simulink library "Lib_LongPRACH"  (R2023b)
settings: Solver=VariableStepAuto  StartTime=0.0  StopTime=10.0  RelTol=1e-3
values from neighbouring files (symbols this model uses):
  prach = waveconfig.PRACH.Config    [hNRPRACHWaveformGenerator.m]
undefined symbols (not defined in the file or in its folder): AdvDSPBChannelOutDisplay, AdvDSPBDMemDisplay, AdvDSPBInDisplay, AdvDSPBOutDisplay, dpoly, dspba, dspba_ChannelInVis, dspba_ChannelOutVis, dspba_internal_get_channel_ports, evalAionMaskParam, latency, latencyCorrection, NTxAnts, primtype, UseDontCare, value
libraries: DSPBAPrim x553, DSPBABase x32, DSPBAFilters x24, DSPBAControl x18, DSPBAModelBus x8, DSPBAWaveformSynth x4, DspbAdvFftLibrary x2, DSPBAUtilities x2
(part 2 of 8)

== system Lib_LongPRACH/prach_wrap/MUX_ConfigId ==
  din0 : Inport
  vin0 : Inport  Port=2  OutDataTypeStr=boolean
  chin0 : Inport  Port=3  OutDataTypeStr=uint8
  SFN : Inport  Port=4
  HFN : Inport  Port=5
  prach_config_index : Inport  Port=6
  4G Config Index : Subsystem
  5G Config Index paired : Subsystem  Commented=on
  5G Config Index unpaired : Subsystem
  And : DSPBAPrim/And  primtype=and  nInputs=2  nOutputs=1  omode=Inherit via internal rule  otype=sfix(16)  scale=2^-15  rndmethod=Unbiased  factor=1  satmethod=Symmetric  shift_vec=[0 1 2 -1]  value=0  inPortNames=[' '; ' '; ' '; ' '; ' '; ' '; ' '; ' '; ' '; ' '; ' '; ' '; ' '; ' '; ' '; ' '; ]  outPortNames=[' ']  dspbaimage=dspba_prim.svg  text=fprintf('&');  style=Optimised  visibilities=8+2  version=20211007
  BitCombine : DSPBAPrim/BitCombine  primtype=bitcombine  nInputs=2  nOutputs=1  omode=Inherit via internal rule  otype=sfix(16)  scale=2^-15  rndmethod=Unbiased  factor=1  satmethod=Symmetric  shift_vec=[0 1 2 -1]  value=0  inPortNames=['l'; 'h';]  outPortNames=[' ']  dspbaimage=dspba_prim.svg  text=fprintf('[h,l]');  style=Optimised  visibilities=8+2  version=20211007
  ChannelIn : DSPBAPrim/ChannelIn  primtype=channelin  nInputs=dspba_internal_get_channel_ports(gcb)  nOutputs=dspba_internal_get_channel_ports(gcb)  omode=Inherit via internal rule  otype=sfix(16)  scale=2^-15  rndmethod=Unbiased  factor=1  satmethod=Symmetric  shift_vec=[0 1 2 -1]  value=1  inPortNames=['v'; 'c'; '0'; '1'; '2'; '3'; '4'; '5'; '6'; '7'; '8'; '9'; 'A'; 'B'; 'D'; 'E'; 'F'; 'G'; 'H'; 'I'; 'J'; 'K'; 'L'; 'M'; 'N'; 'O'; 'P'; 'Q'; 'R'; 'S'; 'T'; 'U'; 'W'; 'X'; 'Y'; 'Z']  outPortNames=['v'; 'c'; '0'; '1'; '2'; '3'; '4'; '5'; '6'; '7'; '8'; '9'; 'A'; 'B'; 'D'; 'E'; 'F'; 'G'; 'H'; 'I'; 'J'; 'K'; 'L'; 'M'; 'N'; 'O'; 'P'; 'Q'; 'R'; 'S'; 'T'; 'U'; 'W'; 'X'; 'Y'; 'Z']  dspbaimage=dspba_prim_channel_tall.svg  text=fprintf('In');  style=Optimised  dataSignals=1  foldingEnabled=off  channels=1  sampleRate=200  packetBeginPresent=off  packetBeginEnabled=off  visibilities=dspba_ChannelInVis(gcb)  latencyCorrection=0  scheduleOrigin=on  version=20211214
  ChannelOut : DSPBAPrim/ChannelOut  primtype=channelout  nInputs=dspba_internal_get_channel_ports(gcb)  nOutputs=dspba_internal_get_channel_ports(gcb)  omode=Inherit via internal rule  otype=sfix(16)  scale=2^-15  rndmethod=Unbiased  factor=1  satmethod=Symmetric  shift_vec=[0 1 2 -1]  value=2  inPortNames=['v'; 'c'; '0'; '1'; '2'; '3'; '4'; '5'; '6'; '7'; '8'; '9'; 'A'; 'B'; 'D'; 'E'; 'F'; 'G'; 'H'; 'I'; 'J'; 'K'; 'L'; 'M'; 'N'; 'O'; 'P'; 'Q'; 'R'; 'S'; 'T'; 'U'; 'W'; 'X'; 'Y'; 'Z']  outPortNames=['v'; 'c'; '0'; '1'; '2'; '3'; '4'; '5'; '6'; '7'; '8'; '9'; 'A'; 'B'; 'D'; 'E'; 'F'; 'G'; 'H'; 'I'; 'J'; 'K'; 'L'; 'M'; 'N'; 'O'; 'P'; 'Q'; 'R'; 'S'; 'T'; 'U'; 'W'; 'X'; 'Y'; 'Z']  dspbaimage=dspba_prim_channel_tall.svg  text=fprintf('Out%s', AdvDSPBChannelOutDisplay(latency));  style=Optimised  dataSignals=2  foldingEnabled=off  channels=1  sampleRate=200  packetBeginPresent=off  packetBeginEnabled=off  visibilities=dspba_ChannelOutVis(gcb)  latency=1  latencyCorrection=0  version=20211214
  Convert2 : DSPBAPrim/Convert  primtype=convert  nInputs=1  nOutputs=1  omode=Specify via dialog  otype=uint(4)  scale=2^0  rndmethod=Truncate  factor=1  satmethod=None  shift_vec=[0 1 2 -1]  value=round([0:255]/17)  inPortNames=[' '; ' ';]  outPortNames=[' '; 'c']  dspbaimage=dspba_prim_wide.svg  text=fprintf('convert');  style=Optimised  visibilities=8+64+256+2^17  clipdetect=off  floatPrecision=float32_m23  advOptions=[]  version=20211007
  GPIn : DSPBAPrim/GPIn  primtype=gpin  nInputs=evalAionMaskParam(gcb,'value',1)  nOutputs=evalAionMaskParam(gcb,'value',1)  omode=Inherit via internal rule  otype=sfix(16)  scale=2^-15  rndmethod=Unbiased  factor=1  satmethod=Symmetric  shift_vec=[0 1 2 -1]  value=1  inPortNames=[' ' ' ' ' ' ' ' ' ' ' ' ' ' ' ' ' ' ' ' ' ' ' ' ' ' ' ' ' ' ' ' ' ' ' ' ' ' ' ' ' ' ' ' ' ' ' ' ' ' ' ' ' ' ' ' ' ' ' ' ' ' ' ' ' ' ' ' ' ']'  outPortNames=[' ' ' ' ' ' ' ' ' ' ' ' ' ' ' ' ' ' ' ' ' ' ' ' ' ' ' ' ' ' ' ' ' ' ' ' ' ' ' ' ' ' ' ' ' ' ' ' ' ' ' ' ' ' ' ' ' ' ' ' ' ' ' ' ' ' ' ' ' ']'  dspbaimage=dspba_prim_channel_tall.svg  text=fprintf('GPIn');  style=Optimised  visibilities=1024  latencyCorrection=0  scheduleOrigin=on  version=20211214
  GPIn1 : DSPBAPrim/GPIn  primtype=gpin  nInputs=evalAionMaskParam(gcb,'value',1)  nOutputs=evalAionMaskParam(gcb,'value',1)  omode=Inherit via internal rule  otype=sfix(16)  scale=2^-15  rndmethod=Unbiased  factor=1  satmethod=Symmetric  shift_vec=[0 1 2 -1]  value=1  inPortNames=[' ' ' ' ' ' ' ' ' ' ' ' ' ' ' ' ' ' ' ' ' ' ' ' ' ' ' ' ' ' ' ' ' ' ' ' ' ' ' ' ' ' ' ' ' ' ' ' ' ' ' ' ' ' ' ' ' ' ' ' ' ' ' ' ' ' ' ' ' ']'  outPortNames=[' ' ' ' ' ' ' ' ' ' ' ' ' ' ' ' ' ' ' ' ' ' ' ' ' ' ' ' ' ' ' ' ' ' ' ' ' ' ' ' ' ' ' ' ' ' ' ' ' ' ' ' ' ' ' ' ' ' ' ' ' ' ' ' ' ' ' ' ' ']'  dspbaimage=dspba_prim_channel_tall.svg  text=fprintf('GPIn');  style=Optimised  visibilities=1024  latencyCorrection=0  scheduleOrigin=on  version=20211214
  GPIn2 : DSPBAPrim/GPIn  primtype=gpin  nInputs=evalAionMaskParam(gcb,'value',1)  nOutputs=evalAionMaskParam(gcb,'value',1)  omode=Inherit via internal rule  otype=sfix(16)  scale=2^-15  rndmethod=Unbiased  factor=1  satmethod=Symmetric  shift_vec=[0 1 2 -1]  value=1  inPortNames=[' ' ' ' ' ' ' ' ' ' ' ' ' ' ' ' ' ' ' ' ' ' ' ' ' ' ' ' ' ' ' ' ' ' ' ' ' ' ' ' ' ' ' ' ' ' ' ' ' ' ' ' ' ' ' ' ' ' ' ' ' ' ' ' ' ' ' ' ' ']'  outPortNames=[' ' ' ' ' ' ' ' ' ' ' ' ' ' ' ' ' ' ' ' ' ' ' ' ' ' ' ' ' ' ' ' ' ' ' ' ' ' ' ' ' ' ' ' ' ' ' ' ' ' ' ' ' ' ' ' ' ' ' ' ' ' ' ' ' ' ' ' ' ']'  dspbaimage=dspba_prim_channel_tall.svg  text=fprintf('GPIn');  style=Optimised  visibilities=1024  latencyCorrection=0  scheduleOrigin=on  version=20211214
  Mux1 : DSPBAPrim/Mux  primtype=mux  nInputs=evalAionMaskParam(gcb,'value',1)+1  nOutputs=1  omode=Inherit via internal rule  otype=sfix(16)  scale=2^-15  rndmethod=Unbiased  factor=1  satmethod=Symmetric  shift_vec=[0 1 2 -1]  value=2  inPortNames=['s '; 'd0'; 'd1'; 'd2'; 'd3'; 'd4'; 'd5'; 'd6'; 'd7'; 'd8'; 'd9';]  outPortNames=[' ']  dspbaimage=dspba_prim_tall.svg  text=fprintf('%s', primtype);  style=Optimised  visibilities=1032  version=20211007
  RegField2 : DSPBAModelBus/RegField  reg_name=MMoffset.prach_technology  reg_rwmode=Read/Write  reg_msb=0  reg_lsb=0  reg_mode=Specify via dialog  reg_type=ufix(1)  reg_scale=2^0  reg_init=prach_technology  reg_desc=4G = 0, 5G = 1 Technology  reg_modal=off  reg_desc0=0  reg_desc1=0  reg_desc2=0  reg_desc3=0  reg_desc4=0  reg_desc5=0  reg_desc6=0  reg_desc7=0  SampleTime=-1  version=20090407
  SynthesisInfo : DSPBAPrim/SynthesisInfo  primtype=synthinfo  nInputs=0  nOutputs=0  omode=Inherit via internal rule  otype=sfix(16)  scale=2^-15  rndmethod=Truncate  factor=1  satmethod=Symmetric  shift_vec=[0 1 2 -1]  value=99  inPortNames=[' '; ' ';]  outPortNames=[' ']  dspbaimage=dspba_prim_ctrl.jpg  text=fprintf('Style=%s', style);  style=Scheduled  visibilities=2^17+2^18+2^19+2^20+2^21+2^22+2^23+2^24  constraintPair=None  constraintRelation=>  constraintLimit=2  modelRefSign=+  modelRef=''  showSchedule=off  simulationMode=Use Global Value  resetMinimization=Conditional - On for ChannelIn/Out only  version=20220106
  dout : Outport  VectorParamsAs1DForOutWhenUnconnected=off
  vout : Outport  Port=2  VectorParamsAs1DForOutWhenUnconnected=off
  cout : Outport  Port=3  VectorParamsAs1DForOutWhenUnconnected=off
  TimeReference : Outport  Port=4  VectorParamsAs1DForOutWhenUnconnected=off
  wires:
  ChannelIn/1 -> And/2
  ChannelOut/1 -> vout/1
  ChannelOut/2 -> cout/1
  ChannelOut/3 -> dout/1
  ChannelIn/2 -> ChannelOut/2
  And/1 -> ChannelOut/1
  SFN/1 -> GPIn1/1
  HFN/1 -> GPIn/1
  prach_config_index/1 -> GPIn2/1
  vin0/1 -> ChannelIn/1
  chin0/1 -> ChannelIn/2
  din0/1 -> ChannelIn/3
  ChannelIn/3 -> ChannelOut/3
  GPIn/1 -> Convert2/1
  Convert2/1 -> BitCombine/1, 5G Config Index unpaired/1(SubFrame), 4G Config Index/3(SubFrame)
  GPIn2/1 -> 4G Config Index/1(ConfigIdx), 5G Config Index unpaired/2(ConfigIdx)
  GPIn1/1 -> BitCombine/2, 5G Config Index unpaired/3(SFN), 4G Config Index/2(SFN)
  5G Config Index unpaired/1(Out2) -> Mux1/3
  Mux1/1 -> And/1
  4G Config Index/1(Out2) -> Mux1/2
  RegField2/1 -> Mux1/1
  BitCombine/1 -> ChannelOut/4
  ChannelOut/4 -> TimeReference/1

== system Lib_LongPRACH/prach_wrap/S2B_FFT ==
  note: FFT
  note: scaling
  din : Inport
  vin : Inport  Port=2
  cin : Inport  Port=3
  Complex to Real-Imag : ComplexToRealImag
  Const6 : DSPBAPrim/Const  primtype=const  nInputs=0  nOutputs=1  omode=Inherit via back propagation  otype=ufix(8)  scale=2^0  rndmethod=Unbiased  factor=1  satmethod=Symmetric  shift_vec=[0 1 2 -1]  value=1  inPortNames=['+'; '+';]  outPortNames=[' ']  dspbaimage=dspba_prim.svg  text=fprintf('%s', num2str(value));  style=Optimised  visibilities=8 + 1024  floatPrecision=float32_m23  warnSaturation=on  version=20211007  SampleTime=inf
  FFT1 : DspbAdvFftLibrary/Common/FFT  IFFT=false  subchannels=1  br_in=true  N=nextpow2(prach.Nfft)  in_type=fixdt(1,16,15)  type_strings=dspba.fft.full_wordgrowth(true, false, nextpow2(prach.Nfft), fixdt(1,16,15), fixdt(1,16,15))  faithful=false
      link override ChannelOut1: nInputs=dspba_internal_get_channel_ports(gcb, 'inputs')  nOutputs=dspba_internal_get_channel_ports(gcb, 'outputs')  value=1  packetBeginEnabled=off  latency=57  version=20140818
  Real-Imag to Complex : RealImagToComplex
  RegField1 : DSPBAModelBus/RegField  Commented=on  reg_name=MMoffset.prach_fft_scale  reg_rwmode=Read/Write  reg_msb=5  reg_lsb=0  reg_mode=Specify via dialog  reg_type=ufix(6)  reg_scale=2^0  reg_init=18  reg_desc=PRACH Sym Extraction Registers  reg_modal=off  reg_desc0=0  reg_desc1=0  reg_desc2=0  reg_desc3=0  reg_desc4=0  reg_desc5=0  reg_desc6=0  reg_desc7=0  SampleTime=-1  version=20090407
  S2B : Subsystem
  Scale : DSPBABase/Scale  otype=sfix(16)  scale=2^-FFT_frac_scaling  rndmethod=Biased  factor=1  satmethod=Symmetric  shift_vec=0  latency=3  simulationMode=Use Global Value  version=20130807
  Scale1 : DSPBABase/Scale  otype=sfix(16)  scale=2^-FFT_frac_scaling  rndmethod=Biased  factor=1  satmethod=Symmetric  shift_vec=0  latency=3  simulationMode=Use Global Value  version=20130807
  Terminator{,1..3} (4 alike) : Terminator
  To Workspace1 : ToWorkspace  VariableName=S2B_dout  SampleTime=-1
  To Workspace2 : ToWorkspace  VariableName=S2B_valid  SampleTime=-1
  To Workspace3 : ToWorkspace  VariableName=S2B_chout  SampleTime=-1
  To Workspace4 : ToWorkspace  VariableName=fftcore_vout  SampleTime=-1
  To Workspace5 : ToWorkspace  VariableName=fftcore_chout  SampleTime=-1
  To Workspace6 : ToWorkspace  VariableName=fftcore_dout  SampleTime=-1
  dout : Outport  VectorParamsAs1DForOutWhenUnconnected=off
  vout : Outport  Port=2  VectorParamsAs1DForOutWhenUnconnected=off
  cout : Outport  Port=3  VectorParamsAs1DForOutWhenUnconnected=off
  wires:
  Real-Imag to Complex/1 -> dout/1
  Scale/2 -> vout/1
  Scale/3 -> cout/1
  din/1 -> S2B/1(data_in)
  vin/1 -> S2B/2(data_valid)
  Scale/4 -> Terminator3/1
  Const6/1 -> Scale/4, Scale1/4
  Scale1/4 -> Terminator2/1
  Scale1/3 -> Terminator1/1
  Scale1/2 -> Terminator/1
  Scale1/1 -> Real-Imag to Complex/2
  FFT1/2 -> To Workspace5/1, Scale/3, Scale1/3
  FFT1/3 -> To Workspace6/1, Complex to Real-Imag/1
  Complex to Real-Imag/2 -> Scale1/1
  Scale/1 -> Real-Imag to Complex/1
  Complex to Real-Imag/1 -> Scale/1
  FFT1/1 -> To Workspace4/1, Scale1/2, Scale/2
  S2B/3(ch_no) -> FFT1/2, To Workspace3/1
  S2B/2(valid_out) -> To Workspace2/1, FFT1/1
  S2B/1(data_out) -> To Workspace1/1, FFT1/3
  cin/1 -> S2B/3(chin)

== system Lib_LongPRACH/prach_wrap/SYM_SELECT ==
  note: rising edge dv required TBD??
  note: prach start point tbd
  din : Inport
  vin : Inport  Port=2
  chin : Inport  Port=3
  TimeRef : Inport  Port=4
  And : DSPBAPrim/And  primtype=and  nInputs=2  nOutputs=1  omode=Inherit via internal rule  otype=sfix(16)  scale=2^-15  rndmethod=Unbiased  factor=1  satmethod=Symmetric  shift_vec=[0 1 2 -1]  value=0  inPortNames=[' '; ' '; ' '; ' '; ' '; ' '; ' '; ' '; ' '; ' '; ' '; ' '; ' '; ' '; ' '; ' '; ]  outPortNames=[' ']  dspbaimage=dspba_prim.svg  text=fprintf('&');  style=Optimised  visibilities=8+2  version=20211007
  And1 : DSPBAPrim/And  primtype=and  nInputs=2  nOutputs=1  omode=Inherit via internal rule  otype=sfix(16)  scale=2^-15  rndmethod=Unbiased  factor=1  satmethod=Symmetric  shift_vec=[0 1 2 -1]  value=0  inPortNames=[' '; ' '; ' '; ' '; ' '; ' '; ' '; ' '; ' '; ' '; ' '; ' '; ' '; ' '; ' '; ' '; ]  outPortNames=[' ']  dspbaimage=dspba_prim.svg  text=fprintf('&');  style=Optimised  visibilities=8+2  version=20211007
  And2 : DSPBAPrim/And  primtype=and  nInputs=2  nOutputs=1  omode=Inherit via internal rule  otype=sfix(16)  scale=2^-15  rndmethod=Unbiased  factor=1  satmethod=Symmetric  shift_vec=[0 1 2 -1]  value=0  inPortNames=[' '; ' '; ' '; ' '; ' '; ' '; ' '; ' '; ' '; ' '; ' '; ' '; ' '; ' '; ' '; ' '; ]  outPortNames=[' ']  dspbaimage=dspba_prim.svg  text=fprintf('&');  style=Optimised  visibilities=8+2  version=20211007
  ChannelIn : DSPBAPrim/ChannelIn  primtype=channelin  nInputs=dspba_internal_get_channel_ports(gcb)  nOutputs=dspba_internal_get_channel_ports(gcb)  omode=Inherit via internal rule  otype=sfix(16)  scale=2^-15  rndmethod=Unbiased  factor=1  satmethod=Symmetric  shift_vec=[0 1 2 -1]  value=2  inPortNames=['v'; 'c'; '0'; '1'; '2'; '3'; '4'; '5'; '6'; '7'; '8'; '9'; 'A'; 'B'; 'D'; 'E'; 'F'; 'G'; 'H'; 'I'; 'J'; 'K'; 'L'; 'M'; 'N'; 'O'; 'P'; 'Q'; 'R'; 'S'; 'T'; 'U'; 'W'; 'X'; 'Y'; 'Z']  outPortNames=['v'; 'c'; '0'; '1'; '2'; '3'; '4'; '5'; '6'; '7'; '8'; '9'; 'A'; 'B'; 'D'; 'E'; 'F'; 'G'; 'H'; 'I'; 'J'; 'K'; 'L'; 'M'; 'N'; 'O'; 'P'; 'Q'; 'R'; 'S'; 'T'; 'U'; 'W'; 'X'; 'Y'; 'Z']  dspbaimage=dspba_prim_channel_tall.svg  text=fprintf('In');  style=Optimised  dataSignals=2  foldingEnabled=off  channels=1  sampleRate=200  packetBeginPresent=off  packetBeginEnabled=off  visibilities=dspba_ChannelInVis(gcb)  latencyCorrection=0  scheduleOrigin=on  version=20211214
  ChannelOut : DSPBAPrim/ChannelOut  primtype=channelout  nInputs=dspba_internal_get_channel_ports(gcb)  nOutputs=dspba_internal_get_channel_ports(gcb)  omode=Inherit via internal rule  otype=sfix(16)  scale=2^-15  rndmethod=Unbiased  factor=1  satmethod=Symmetric  shift_vec=[0 1 2 -1]  value=2  inPortNames=['v'; 'c'; '0'; '1'; '2'; '3'; '4'; '5'; '6'; '7'; '8'; '9'; 'A'; 'B'; 'D'; 'E'; 'F'; 'G'; 'H'; 'I'; 'J'; 'K'; 'L'; 'M'; 'N'; 'O'; 'P'; 'Q'; 'R'; 'S'; 'T'; 'U'; 'W'; 'X'; 'Y'; 'Z']  outPortNames=['v'; 'c'; '0'; '1'; '2'; '3'; '4'; '5'; '6'; '7'; '8'; '9'; 'A'; 'B'; 'D'; 'E'; 'F'; 'G'; 'H'; 'I'; 'J'; 'K'; 'L'; 'M'; 'N'; 'O'; 'P'; 'Q'; 'R'; 'S'; 'T'; 'U'; 'W'; 'X'; 'Y'; 'Z']  dspbaimage=dspba_prim_channel_tall.svg  text=fprintf('Out%s', AdvDSPBChannelOutDisplay(latency));  style=Optimised  dataSignals=2  foldingEnabled=off  channels=1  sampleRate=200  packetBeginPresent=off  packetBeginEnabled=off  visibilities=dspba_ChannelOutVis(gcb)  latency=3  latencyCorrection=0  version=20211214
  CmpEQ : DSPBAPrim/CmpEQ  primtype=cmpeq  nInputs=2  nOutputs=1  omode=boolean  otype=sfix(16)  scale=2^-15  rndmethod=Unbiased  factor=1  satmethod=Symmetric  shift_vec=[0 1 2 -1]  value=0  inPortNames=[' '; ' ';]  outPortNames=[' ']  dspbaimage=dspba_prim.svg  text=fprintf('==');  style=Optimised  visibilities=0  advOptions=[]  version=20211007
  CmpGE : DSPBAPrim/CmpGE  primtype=cmpgte  nInputs=2  nOutputs=1  omode=boolean  otype=sfix(16)  scale=2^-15  rndmethod=Unbiased  factor=1  satmethod=Symmetric  shift_vec=[0 1 2 -1]  value=0  inPortNames=['a'; 'b';]  outPortNames=[' ']  dspbaimage=dspba_prim.svg  text=fprintf('a>=b');  style=Optimised  visibilities=0  advOptions=[]  version=20211007
  CmpLT : DSPBAPrim/CmpLT  primtype=cmplt  nInputs=2  nOutputs=1  omode=boolean  otype=sfix(16)  scale=2^-15  rndmethod=Unbiased  factor=1  satmethod=Symmetric  shift_vec=[0 1 2 -1]  value=0  inPortNames=['a'; 'b';]  outPortNames=[' ']  dspbaimage=dspba_prim.svg  text=fprintf('a<b');  style=Optimised  visibilities=0  advOptions=[]  version=20211007
  Const2 : DSPBAPrim/Const  primtype=const  nInputs=0  nOutputs=1  omode=Specify via dialog  otype=ufix(1)  scale=2^-0  rndmethod=Unbiased  factor=1  satmethod=Symmetric  shift_vec=[0 1 2 -1]  value=0  inPortNames=['+'; '+';]  outPortNames=[' ']  dspbaimage=dspba_prim.svg  text=fprintf('%s', num2str(value));  style=Optimised  visibilities=8 + 1024  floatPrecision=float32_m23  warnSaturation=on  version=20211007  SampleTime=inf
  Counter : DSPBAPrim/Counter  primtype=counter  nInputs=1  nOutputs=1  omode=Inherit via internal rule  otype=ufix(16)  scale=2^-0  rndmethod=Unbiased  factor=1  satmethod=Symmetric  shift_vec=[0 1 2 -1]  value=[prach.Nfft-1 prach.Nfft 1]  inPortNames=[' '; ' ';]  outPortNames=[' ']  dspbaimage=dspba_prim.svg  text=fprintf('counter\n[%d %d %d]', value(1), value(2), value(3));  style=Optimised  visibilities=8 + 1024  version=20211007
  RegField1 : DSPBAModelBus/RegField  reg_name=MMoffset.prach_out_start  reg_rwmode=Read/Write  reg_msb=15  reg_lsb=0  reg_mode=Specify via dialog  reg_type=ufix(16)  reg_scale=2^0  reg_init=prach.SCstart-1  reg_desc=PRACH Sym Extraction Registers  reg_modal=off  reg_desc0=0  reg_desc1=0  reg_desc2=0  reg_desc3=0  reg_desc4=0  reg_desc5=0  reg_desc6=0  reg_desc7=0  SampleTime=-1  version=20090407
  RegField2 : DSPBAModelBus/RegField  reg_name=MMoffset.prach_out_end  reg_rwmode=Read/Write  reg_msb=15  reg_lsb=0  reg_mode=Specify via dialog  reg_type=ufix(16)  reg_scale=2^0  reg_init=prach.SCend  reg_desc=PRACH Sym Extraction Registers  reg_modal=off  reg_desc0=0  reg_desc1=0  reg_desc2=0  reg_desc3=0  reg_desc4=0  reg_desc5=0  reg_desc6=0  reg_desc7=0  SampleTime=-1  version=20090407
  SynthesisInfo : DSPBAPrim/SynthesisInfo  primtype=synthinfo  nInputs=0  nOutputs=0  omode=Inherit via internal rule  otype=sfix(16)  scale=2^-15  rndmethod=Truncate  factor=1  satmethod=Symmetric  shift_vec=[0 1 2 -1]  value=99  inPortNames=[' '; ' ';]  outPortNames=[' ']  dspbaimage=dspba_prim_ctrl.jpg  text=fprintf('Style=%s', style);  style=Scheduled  visibilities=2^17+2^18+2^19+2^20+2^21+2^22+2^23+2^24  constraintPair=None  constraintRelation=>  constraintLimit=2  modelRefSign=+  modelRef=''  showSchedule=off  simulationMode=Use Global Value  resetMinimization=Conditional - On for ChannelIn/Out only  version=20220106
  To Workspace12 : ToWorkspace  VariableName=prach_cout  SampleTime=-1
  To Workspace7 : ToWorkspace  VariableName=prach_vout  SampleTime=-1
  To Workspace8 : ToWorkspace  VariableName=prach_dout  SampleTime=-1
  Zero_insertion : Subsystem
  latch_0L : DSPBAControl/latch_0L
  dout : Outport  VectorParamsAs1DForOutWhenUnconnected=off
  vout : Outport  Port=2  VectorParamsAs1DForOutWhenUnconnected=off
  cout : Outport  Port=3  VectorParamsAs1DForOutWhenUnconnected=off
  TimeReference : Outport  Port=4  VectorParamsAs1DForOutWhenUnconnected=off
  wires:
  RegField2/1 -> CmpLT/2
  RegField1/1 -> CmpGE/2
  Counter/1 -> CmpLT/1, CmpGE/1
  ChannelIn/1 -> And/1, Counter/1
  ChannelOut/1 -> To Workspace7/1, vout/1
  ChannelOut/2 -> To Workspace12/1, cout/1
  ChannelOut/3 -> dout/1, To Workspace8/1
  din/1 -> ChannelIn/3
  chin/1 -> ChannelIn/2
  vin/1 -> ChannelIn/1
  CmpGE/1 -> And2/1
  CmpLT/1 -> And2/2
  And2/1 -> And/2
  And/1 -> Zero_insertion/1(valid_in), And1/1
  TimeRef/1 -> ChannelIn/4
  ChannelOut/4 -> TimeReference/1
  ChannelIn/4 -> latch_0L/2
  ChannelIn/2 -> Zero_insertion/2(chin), CmpEQ/1
  Const2/1 -> CmpEQ/2
  CmpEQ/1 -> And1/2
  And1/1 -> latch_0L/1
  latch_0L/1 -> ChannelOut/4
  Zero_insertion/3(dataout) -> ChannelOut/3
  Zero_insertion/1(valid_out) -> ChannelOut/1
  Zero_insertion/2("chout ") -> ChannelOut/2
  ChannelIn/3 -> Zero_insertion/3(datain)

== system Lib_LongPRACH/Longprach_C_M_plane/LongPRACH_core/CP_REMOVAL ==
  din : Inport
  vin : Inport  Port=2
  cin : Inport  Port=3
  cp_start : Inport  Port=4
  gt_end : Inport  Port=5
  filt_flush_en : Inport  Port=6
  RemoveCP5 : Subsystem
  dout : Outport  VectorParamsAs1DForOutWhenUnconnected=off
  vout : Outport  Port=2  VectorParamsAs1DForOutWhenUnconnected=off
  cout : Outport  Port=3  VectorParamsAs1DForOutWhenUnconnected=off
  filt_flush : Outport  Port=4
  sync_out : Outport  Port=5
  wires:
  vin/1 -> RemoveCP5/1(vin)
  cin/1 -> RemoveCP5/2(chin)
  din/1 -> RemoveCP5/3(din)
  RemoveCP5/1(vout) -> vout/1
  RemoveCP5/2(cout) -> cout/1
  RemoveCP5/3(dout) -> dout/1
  cp_start/1 -> RemoveCP5/4(cp_start)
  gt_end/1 -> RemoveCP5/5(gt_end)
  RemoveCP5/4(filt_flush) -> filt_flush/1
  filt_flush_en/1 -> RemoveCP5/6(filt_flush_en)
  RemoveCP5/5(sync_out) -> sync_out/1

== system Lib_LongPRACH/Longprach_C_M_plane/LongPRACH_core/DECIMATION1 ==
  din : Inport
  vin : Inport  Port=2
  cin : Inport  Port=3
  filt_flush : Inport  Port=4
  Stage1 : Subsystem
  Stage2 : Subsystem
  Stage3 : Subsystem
  Stage5 : Subsystem
  Stage6 : Subsystem
  stage4 : Subsystem
  dout : Outport  VectorParamsAs1DForOutWhenUnconnected=off
  vout : Outport  Port=2  VectorParamsAs1DForOutWhenUnconnected=off
  cout : Outport  Port=3  VectorParamsAs1DForOutWhenUnconnected=off
  wires:
  filt_flush/1 -> Stage1/4(flush_en), Stage6/4(flush_en)
  cin/1 -> Stage1/3(ch_in)
  Stage2/1(data_out) -> Stage3/1(data_in)
  din/1 -> Stage1/1(data_in)
  Stage1/1(data_out) -> Stage2/1(data_in)
  Stage1/3(ch_out) -> Stage2/3(ch_in)
  Stage6/3(ch_out) -> cout/1
  Stage2/2(valid_out) -> Stage3/2(valid_in)
  stage4/3(ch_out) -> Stage5/3(ch_in)
  vin/1 -> Stage1/2(valid_in)
  Stage6/1(data_out) -> dout/1
  Stage1/2(valid_out) -> Stage2/2(valid_in)
  stage4/2(valid_out) -> Stage5/2(valid_in)
  Stage5/3(ch_out) -> Stage6/3(ch_in)
  Stage5/2(valid_out) -> Stage6/2(valid_in)
  Stage5/1(data_out) -> Stage6/1(data_in)
  Stage2/3(ch_out) -> Stage3/3(ch_in)
  stage4/1(data_out) -> Stage5/1(data_in)
  Stage3/3(ch_out) -> stage4/3(ch_in)
  Stage3/2(valid_out) -> stage4/2(valid_in)
  Stage6/2(valid_out) -> vout/1
  Stage3/1(data_out) -> stage4/1(data_in)

== system Lib_LongPRACH/Longprach_C_M_plane/LongPRACH_core/FFTShift ==
  data_in : Inport
  data_valid : Inport  Port=2
  chin : Inport  Port=3
  ChNoLatch : Subsystem  Commented=on
  ChannelIn : DSPBAPrim/ChannelIn  primtype=channelin  nInputs=dspba_internal_get_channel_ports(gcb)  nOutputs=dspba_internal_get_channel_ports(gcb)  omode=Inherit via internal rule  otype=sfix(16)  scale=2^-15  rndmethod=Unbiased  factor=1  satmethod=Symmetric  shift_vec=[0 1 2 -1]  value=1  inPortNames=['v'; 'c'; '0'; '1'; '2'; '3'; '4'; '5'; '6'; '7'; '8'; '9'; 'A'; 'B'; 'D'; 'E'; 'F'; 'G'; 'H'; 'I'; 'J'; 'K'; 'L'; 'M'; 'N'; 'O'; 'P'; 'Q'; 'R'; 'S'; 'T'; 'U'; 'W'; 'X'; 'Y'; 'Z']  outPortNames=['v'; 'c'; '0'; '1'; '2'; '3'; '4'; '5'; '6'; '7'; '8'; '9'; 'A'; 'B'; 'D'; 'E'; 'F'; 'G'; 'H'; 'I'; 'J'; 'K'; 'L'; 'M'; 'N'; 'O'; 'P'; 'Q'; 'R'; 'S'; 'T'; 'U'; 'W'; 'X'; 'Y'; 'Z']  dspbaimage=dspba_prim_channel_tall.svg  text=fprintf('In');  style=Optimised  dataSignals=1  foldingEnabled=off  channels=1  sampleRate=200  packetBeginPresent=off  packetBeginEnabled=off  visibilities=dspba_ChannelInVis(gcb)  latencyCorrection=0  scheduleOrigin=on  version=20211214
  ChannelOut : DSPBAPrim/ChannelOut  primtype=channelout  nInputs=dspba_internal_get_channel_ports(gcb)  nOutputs=dspba_internal_get_channel_ports(gcb)  omode=Inherit via internal rule  otype=sfix(16)  scale=2^-15  rndmethod=Unbiased  factor=1  satmethod=Symmetric  shift_vec=[0 1 2 -1]  value=1  inPortNames=['v'; 'c'; '0'; '1'; '2'; '3'; '4'; '5'; '6'; '7'; '8'; '9'; 'A'; 'B'; 'D'; 'E'; 'F'; 'G'; 'H'; 'I'; 'J'; 'K'; 'L'; 'M'; 'N'; 'O'; 'P'; 'Q'; 'R'; 'S'; 'T'; 'U'; 'W'; 'X'; 'Y'; 'Z']  outPortNames=['v'; 'c'; '0'; '1'; '2'; '3'; '4'; '5'; '6'; '7'; '8'; '9'; 'A'; 'B'; 'D'; 'E'; 'F'; 'G'; 'H'; 'I'; 'J'; 'K'; 'L'; 'M'; 'N'; 'O'; 'P'; 'Q'; 'R'; 'S'; 'T'; 'U'; 'W'; 'X'; 'Y'; 'Z']  dspbaimage=dspba_prim_channel_tall.svg  text=fprintf('Out%s', AdvDSPBChannelOutDisplay(latency));  style=Optimised  dataSignals=1  foldingEnabled=off  channels=1  sampleRate=200  packetBeginPresent=off  packetBeginEnabled=off  visibilities=dspba_ChannelOutVis(gcb)  latency=4  latencyCorrection=0  version=20211214
  DualMem : DSPBAPrim/DualMem  primtype=dualmem  nInputs=4  nOutputs=2  omode=Inherit via internal rule  otype=sfix(16)  scale=2^-15  rndmethod=Unbiased  factor=1  satmethod=Symmetric  shift_vec=[0 1 2 -1]  value=[zeros(1024*2, 1)]  inPortNames=['d1'; 'a1'; 'w1'; 'd2'; 'a2'; 'w2']  outPortNames=['q1'; 'q2']  dspbaimage=dspba_prim_tall.svg  text=fprintf('dmem%s',AdvDSPBDMemDisplay(UseDontCare));  style=Optimised  visibilities=8 + 1024 + 2^17 + 2^18  UseDontCare=on  TwinWritePorts=off  init=on  ProvideReadAccess=off  version=20211007
  Mem_rd_wr : Subsystem
  Subsystem : Subsystem
  SynthesisInfo : DSPBAPrim/SynthesisInfo  primtype=synthinfo  nInputs=0  nOutputs=0  omode=Inherit via internal rule  otype=sfix(16)  scale=2^-15  rndmethod=Truncate  factor=1  satmethod=Symmetric  shift_vec=[0 1 2 -1]  value=99  inPortNames=[' '; ' ';]  outPortNames=[' ']  dspbaimage=dspba_prim_ctrl.jpg  text=fprintf('Style=%s', style);  style=Scheduled  visibilities=2^17+2^18+2^19+2^20+2^21+2^22+2^23+2^24  constraintPair=None  constraintRelation=>  constraintLimit=2  modelRefSign=+  modelRef=''  showSchedule=off  simulationMode=Use Global Value  resetMinimization=Conditional - On for ChannelIn/Out only  version=20220106
  Terminator : Terminator
  data_out : Outport
  valid_out : Outport  Port=2
  ch_no : Outport  Port=3
  wires:
  Subsystem/1(q) -> ChannelOut/2
  ChannelIn/2 -> Subsystem/2(d)
  Mem_rd_wr/5(wba) -> Subsystem/1(toggleline)
  ChannelOut/2 -> ch_no/1
  Mem_rd_wr/4(rd_validout) -> ChannelOut/1
  ChannelOut/1 -> valid_out/1
  DualMem/2 -> ChannelOut/3
  ChannelOut/3 -> data_out/1
  chin/1 -> ChannelIn/2
  data_valid/1 -> ChannelIn/1
  ChannelIn/1 -> Mem_rd_wr/1(valid)
  data_in/1 -> ChannelIn/3
  ChannelIn/3 -> DualMem/1
  Mem_rd_wr/3(rd_addr_final) -> DualMem/4
  DualMem/1 -> Terminator/1
  Mem_rd_wr/1(Wr_addr_final) -> DualMem/2
  Mem_rd_wr/2(We) -> DualMem/3

== system Lib_LongPRACH/Longprach_C_M_plane/LongPRACH_core/MIXER ==
  note: mixer
  din : Inport
  vin : Inport  Port=2
  chin : Inport  Port=3
  sync : Inport  Port=4
  Complex to Real-Imag1 : ComplexToRealImag
  ComplexMixer1 : DSPBAWaveformSynth/ComplexMixer  nInputRate=prach.SampleRateMSPS  nchan=prach.no_of_chan/2  nfreq=NTxAnts  latency=6  simulationMode=Use Global Value  version=20090407
  Const1 : DSPBAPrim/Const  primtype=const  nInputs=0  nOutputs=1  omode=Inherit via back propagation  otype=ufix(8)  scale=2^0  rndmethod=Unbiased  factor=1  satmethod=Symmetric  shift_vec=[0 1 2 -1]  value=1  inPortNames=['+'; '+';]  outPortNames=[' ']  dspbaimage=dspba_prim.svg  text=fprintf('%s', num2str(value));  style=Optimised  visibilities=8 + 1024  floatPrecision=float32_m23  warnSaturation=on  version=20211007  SampleTime=inf
  Const2 : DSPBAPrim/Const  primtype=const  nInputs=0  nOutputs=1  omode=boolean  otype=uint(30)  scale=2^0  rndmethod=Unbiased  factor=1  satmethod=Symmetric  shift_vec=[0 1 2 -1]  value=0  inPortNames=['+'; '+';]  outPortNames=[' ']  dspbaimage=dspba_prim.svg  text=fprintf('%s', num2str(value));  style=Optimised  visibilities=8 + 1024  floatPrecision=float32_m23  warnSaturation=on  version=20211007  SampleTime=inf
  Const6 : DSPBAPrim/Const  primtype=const  nInputs=0  nOutputs=1  omode=Specify via dialog  otype=uint(30)  scale=2^0  rndmethod=Unbiased  factor=1  satmethod=Symmetric  shift_vec=[0 1 2 -1]  value=0  inPortNames=['+'; '+';]  outPortNames=[' ']  dspbaimage=dspba_prim.svg  text=fprintf('%s', num2str(value));  style=Optimised  visibilities=8 + 1024  floatPrecision=float32_m23  warnSaturation=on  version=20211007  SampleTime=inf
  NCO1 : DSPBAWaveformSynth/NCO  outputRate=prach.SampleRateMSPS  otype=sfix(18)  scale=2^-17  accumBitWidth=30  phaseIncrAndInv=ones(1,NTxAnts) *prach.NCO  phaseIncrAndInvMap=MMoffset.NCO  rwmode=Read/Write  exposebus=off  version=20090407  SampleTime=-1  expSFDR=108.36  accumPrecision=+/- 0.05722  phaseIncrInMHz="[48.615  48.615  48.615  48.615]"  outWidth=3  tableSize=8  latency=17
      settings: AttributesFormatString=%<latency>
  Real-Imag to Complex : RealImagToComplex
  Real-Imag to Complex1 : RealImagToComplex
  SampleDelay : DSPBAPrim/SampleDelay  primtype=sampdelay  nInputs=1  nOutputs=1  omode=Inherit via internal rule  otype=sfix(16)  scale=2^-15  rndmethod=Unbiased  factor=1  satmethod=Symmetric  shift_vec=[0 1 2 -1]  floatPrecision=float32_m23  value=1  inPortNames=[' '; ' ';]  outPortNames=[' ']  dspbaimage=dspba_prim.svg  text=dpoly(1, eye(1,value+1), 'z')  style=Optimised  visibilities=8 + 1024 + 2^17 + 2^18  flexible=off  slackgroup=0  augmented=0  version=20211007  advOptions=[]
  SampleDelay1 : DSPBAPrim/SampleDelay  primtype=sampdelay  nInputs=1  nOutputs=1  omode=Inherit via internal rule  otype=sfix(16)  scale=2^-15  rndmethod=Unbiased  factor=1  satmethod=Symmetric  shift_vec=[0 1 2 -1]  floatPrecision=float32_m23  value=1  inPortNames=[' '; ' ';]  outPortNames=[' ']  dspbaimage=dspba_prim.svg  text=dpoly(1, eye(1,value+1), 'z')  style=Optimised  visibilities=8 + 1024 + 2^17 + 2^18  flexible=off  slackgroup=0  augmented=0  version=20211007  advOptions=[]
  Scale : DSPBABase/Scale  otype=sfix(16)  scale=2^-15  rndmethod=Biased  factor=1  satmethod=Symmetric  shift_vec=0  latency=2  simulationMode=Use Global Value  version=20130807
  Scale1 : DSPBABase/Scale  otype=sfix(16)  scale=2^-15  rndmethod=Biased  factor=1  satmethod=Symmetric  shift_vec=0  latency=2  simulationMode=Use Global Value  version=20130807
  Terminator{,1..7} (8 alike) : Terminator
  To Workspace1 : ToWorkspace  VariableName=NCO_valid  SampleTime=-1
  To Workspace5 : ToWorkspace  VariableName=NCO_dout  SampleTime=-1
  delay_FIFO : DSPBAPrim/FIFO  primtype=fifo  nInputs=3  nOutputs=4  omode=Inherit via internal rule  otype=sfix(16)  scale=2^-15  rndmethod=Unbiased  factor=1  satmethod=Symmetric  shift_vec=[0 1 2 -1]  value=[32 4 16]  inPortNames=['w'; 'd'; 'r'; 'f']  outPortNames=['v'; 'q'; 't'; 'f']  dspbaimage=dspba_prim_tall.svg  text=fprintf('fifo');  style=Optimised  visibilities=263168  version=20211007  user_sclr=off
  output4 : Scope  NumInputPorts=5
  dout : Outport  VectorParamsAs1DForOutWhenUnconnected=off
  vout : Outport  Port=2  VectorParamsAs1DForOutWhenUnconnected=off
  cout : Outport  Port=3  VectorParamsAs1DForOutWhenUnconnected=off
  wires:
  Const2/1 -> NCO1/4
  Real-Imag to Complex1/1 -> To Workspace5/1
  SampleDelay1/1 -> NCO1/1
  SampleDelay/1 -> NCO1/2
  Scale/4 -> Terminator4/1
  ComplexMixer1/4 -> Scale/3, Scale1/3
  NCO1/3 -> output4/2, ComplexMixer1/3, delay_FIFO/3, To Workspace1/1
  NCO1/1 -> Real-Imag to Complex1/2, ComplexMixer1/5, output4/4
  Const1/1 -> Scale/4, Scale1/4
  Complex to Real-Imag1/2 -> ComplexMixer1/2
  delay_FIFO/2 -> Complex to Real-Imag1/1
  NCO1/4 -> ComplexMixer1/4, output4/3
  Complex to Real-Imag1/1 -> ComplexMixer1/1
  ComplexMixer1/3 -> Scale/2, Scale1/2
  NCO1/2 -> ComplexMixer1/6, output4/5, Real-Imag to Complex1/1
  ComplexMixer1/2 -> Scale1/1
  ComplexMixer1/1 -> Scale/1
  Scale1/1 -> Real-Imag to Complex/2
  Scale/1 -> Real-Imag to Complex/1
  Scale1/3 -> Terminator6/1
  Scale1/2 -> Terminator5/1
  Scale1/4 -> Terminator3/1
  delay_FIFO/4 -> Terminator1/1
  delay_FIFO/3 -> Terminator2/1
  delay_FIFO/1 -> Terminator/1
  Scale/3 -> cout/1
  Const6/1 -> NCO1/3
  din/1 -> delay_FIFO/2
  chin/1 -> SampleDelay1/1
  vin/1 -> SampleDelay/1, output4/1, delay_FIFO/1
  Scale/2 -> vout/1
  Real-Imag to Complex/1 -> dout/1
  sync/1 -> Terminator7/1

== system Lib_LongPRACH/Longprach_C_M_plane/LongPRACH_core/S2B_FFT ==
  note: scaling
  note: FFT
  din : Inport
  vin : Inport  Port=2
  cin : Inport  Port=3
  resetin : Inport  Port=4
  gainin : Inport  Port=5
  Complex to Real-Imag : ComplexToRealImag
  Const6 : DSPBAPrim/Const  primtype=const  nInputs=0  nOutputs=1  omode=Inherit via back propagation  otype=ufix(8)  scale=2^0  rndmethod=Unbiased  factor=1  satmethod=Symmetric  shift_vec=[0 1 2 -1]  value=1  inPortNames=['+'; '+';]  outPortNames=[' ']  dspbaimage=dspba_prim.svg  text=fprintf('%s', num2str(value));  style=Optimised  visibilities=8 + 1024  floatPrecision=float32_m23  warnSaturation=on  version=20211007  SampleTime=inf
  FFT1 : DspbAdvFftLibrary/Common/FFT  IFFT=false  subchannels=1  br_in=true  N=nextpow2(prach.Nfft)  in_type=fixdt(1,16,15)  type_strings=dspba.fft.full_wordgrowth(true, false, nextpow2(prach.Nfft), fixdt(1,16,15), fixdt(1,16,15))  faithful=false
      link override ChannelOut1: nInputs=dspba_internal_get_channel_ports(gcb, 'inputs')  nOutputs=dspba_internal_get_channel_ports(gcb, 'outputs')  value=1  packetBeginEnabled=off  latency=50  version=20140818
  Real-Imag to Complex : RealImagToComplex
  RegField1 : DSPBAModelBus/RegField  Commented=on  reg_name=MMoffset.prach_fft_scale  reg_rwmode=Read/Write  reg_msb=5  reg_lsb=0  reg_mode=Specify via dialog  reg_type=ufix(6)  reg_scale=2^0  reg_init=18  reg_desc=PRACH Sym Extraction Registers  reg_modal=off  reg_desc0=0  reg_desc1=0  reg_desc2=0  reg_desc3=0  reg_desc4=0  reg_desc5=0  reg_desc6=0  reg_desc7=0  SampleTime=-1  version=20090407
  S2B : Subsystem
  Scale : DSPBABase/Scale  otype=sfix(16)  scale=2^-FFT_frac_scaling  rndmethod=Biased  factor=1  satmethod=Symmetric  shift_vec=0  latency=2  simulationMode=Use Global Value  version=20130807
  Scale1 : DSPBABase/Scale  otype=sfix(16)  scale=2^-FFT_frac_scaling  rndmethod=Biased  factor=1  satmethod=Symmetric  shift_vec=0  latency=2  simulationMode=Use Global Value  version=20130807
  Terminator{,1..3} (4 alike) : Terminator
  To Workspace1 : ToWorkspace  VariableName=S2B_dout  SampleTime=-1
  To Workspace2 : ToWorkspace  VariableName=S2B_valid  SampleTime=-1
  To Workspace3 : ToWorkspace  VariableName=S2B_chout  SampleTime=-1
  To Workspace4 : ToWorkspace  VariableName=fftcore_vout  SampleTime=-1
  To Workspace5 : ToWorkspace  VariableName=fftcore_chout  SampleTime=-1
  To Workspace6 : ToWorkspace  VariableName=fftcore_dout  SampleTime=-1
  gain : Subsystem
  dout : Outport  VectorParamsAs1DForOutWhenUnconnected=off
  vout : Outport  Port=2  VectorParamsAs1DForOutWhenUnconnected=off
  cout : Outport  Port=3  VectorParamsAs1DForOutWhenUnconnected=off
  wires:
  cin/1 -> S2B/3(chin)
  S2B/1(data_out) -> gain/1(data_in)
  S2B/2(valid_out) -> gain/2(data_valid)
  S2B/3(ch_no) -> gain/3(chin)
  FFT1/1 -> Scale/2, Scale1/2, To Workspace4/1
  Complex to Real-Imag/1 -> Scale/1
  Scale/1 -> Real-Imag to Complex/1
  Complex to Real-Imag/2 -> Scale1/1
  FFT1/3 -> Complex to Real-Imag/1, To Workspace6/1
  FFT1/2 -> Scale1/3, Scale/3, To Workspace5/1
  Scale1/1 -> Real-Imag to Complex/2
  Scale1/2 -> Terminator/1
  Scale1/3 -> Terminator1/1
  Scale1/4 -> Terminator2/1
  Const6/1 -> Scale1/4, Scale/4
  Scale/4 -> Terminator3/1
  vin/1 -> S2B/2(data_valid)
  din/1 -> S2B/1(data_in)
  Scale/3 -> cout/1
  Scale/2 -> vout/1
  Real-Imag to Complex/1 -> dout/1
  resetin/1 -> S2B/4(resetin)
  gain/1(data_out) -> To Workspace1/1, FFT1/3
  gain/2(valid_out) -> To Workspace2/1, FFT1/1
  gain/3(ch_no) -> To Workspace3/1, FFT1/2
  gainin/1 -> gain/4(gain)

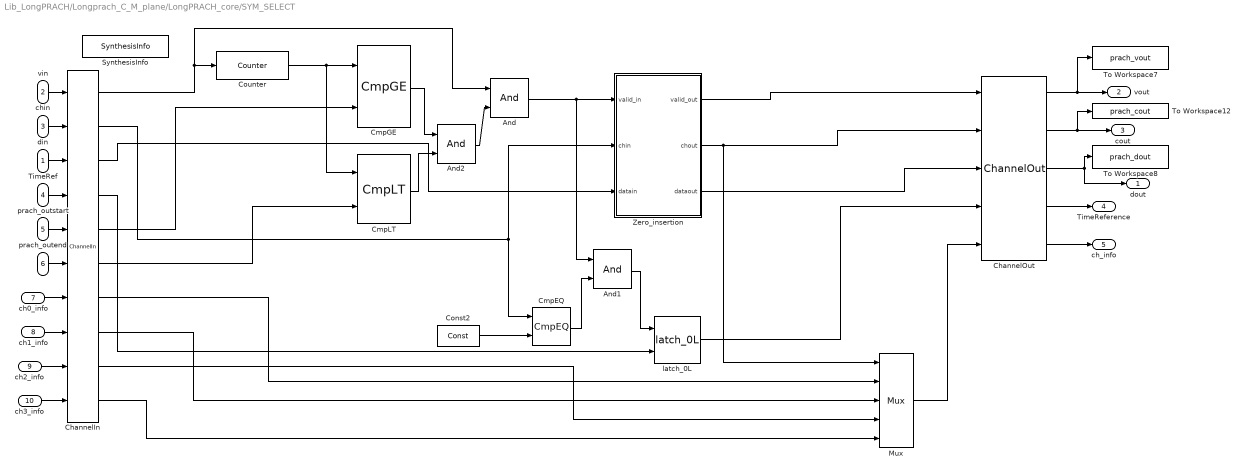
== system Lib_LongPRACH/Longprach_C_M_plane/LongPRACH_core/SYM_SELECT ==
  din : Inport
  vin : Inport  Port=2
  chin : Inport  Port=3
  TimeRef : Inport  Port=4
  prach_outstart : Inport  Port=5
  prach_outend : Inport  Port=6
  ch0_info : Inport  Port=7
  ch1_info : Inport  Port=8
  ch2_info : Inport  Port=9
  ch3_info : Inport  Port=10
  And : DSPBAPrim/And  primtype=and  nInputs=2  nOutputs=1  omode=Inherit via internal rule  otype=sfix(16)  scale=2^-15  rndmethod=Unbiased  factor=1  satmethod=Symmetric  shift_vec=[0 1 2 -1]  value=0  inPortNames=[' '; ' '; ' '; ' '; ' '; ' '; ' '; ' '; ' '; ' '; ' '; ' '; ' '; ' '; ' '; ' '; ]  outPortNames=[' ']  dspbaimage=dspba_prim.svg  text=fprintf('&');  style=Optimised  visibilities=8+2  version=20211007
  And1 : DSPBAPrim/And  primtype=and  nInputs=2  nOutputs=1  omode=Inherit via internal rule  otype=sfix(16)  scale=2^-15  rndmethod=Unbiased  factor=1  satmethod=Symmetric  shift_vec=[0 1 2 -1]  value=0  inPortNames=[' '; ' '; ' '; ' '; ' '; ' '; ' '; ' '; ' '; ' '; ' '; ' '; ' '; ' '; ' '; ' '; ]  outPortNames=[' ']  dspbaimage=dspba_prim.svg  text=fprintf('&');  style=Optimised  visibilities=8+2  version=20211007
  And2 : DSPBAPrim/And  primtype=and  nInputs=2  nOutputs=1  omode=Inherit via internal rule  otype=sfix(16)  scale=2^-15  rndmethod=Unbiased  factor=1  satmethod=Symmetric  shift_vec=[0 1 2 -1]  value=0  inPortNames=[' '; ' '; ' '; ' '; ' '; ' '; ' '; ' '; ' '; ' '; ' '; ' '; ' '; ' '; ' '; ' '; ]  outPortNames=[' ']  dspbaimage=dspba_prim.svg  text=fprintf('&');  style=Optimised  visibilities=8+2  version=20211007
  ChannelIn : DSPBAPrim/ChannelIn  primtype=channelin  nInputs=dspba_internal_get_channel_ports(gcb)  nOutputs=dspba_internal_get_channel_ports(gcb)  omode=Inherit via internal rule  otype=sfix(16)  scale=2^-15  rndmethod=Unbiased  factor=1  satmethod=Symmetric  shift_vec=[0 1 2 -1]  value=8  inPortNames=['v'; 'c'; '0'; '1'; '2'; '3'; '4'; '5'; '6'; '7'; '8'; '9'; 'A'; 'B'; 'D'; 'E'; 'F'; 'G'; 'H'; 'I'; 'J'; 'K'; 'L'; 'M'; 'N'; 'O'; 'P'; 'Q'; 'R'; 'S'; 'T'; 'U'; 'W'; 'X'; 'Y'; 'Z']  outPortNames=['v'; 'c'; '0'; '1'; '2'; '3'; '4'; '5'; '6'; '7'; '8'; '9'; 'A'; 'B'; 'D'; 'E'; 'F'; 'G'; 'H'; 'I'; 'J'; 'K'; 'L'; 'M'; 'N'; 'O'; 'P'; 'Q'; 'R'; 'S'; 'T'; 'U'; 'W'; 'X'; 'Y'; 'Z']  dspbaimage=dspba_prim_channel_tall.svg  text=fprintf('In');  style=Optimised  dataSignals=8  foldingEnabled=off  channels=1  sampleRate=200  packetBeginPresent=off  packetBeginEnabled=off  visibilities=dspba_ChannelInVis(gcb)  latencyCorrection=0  scheduleOrigin=on  version=20211214
  ChannelOut : DSPBAPrim/ChannelOut  primtype=channelout  nInputs=dspba_internal_get_channel_ports(gcb)  nOutputs=dspba_internal_get_channel_ports(gcb)  omode=Inherit via internal rule  otype=sfix(16)  scale=2^-15  rndmethod=Unbiased  factor=1  satmethod=Symmetric  shift_vec=[0 1 2 -1]  value=3  inPortNames=['v'; 'c'; '0'; '1'; '2'; '3'; '4'; '5'; '6'; '7'; '8'; '9'; 'A'; 'B'; 'D'; 'E'; 'F'; 'G'; 'H'; 'I'; 'J'; 'K'; 'L'; 'M'; 'N'; 'O'; 'P'; 'Q'; 'R'; 'S'; 'T'; 'U'; 'W'; 'X'; 'Y'; 'Z']  outPortNames=['v'; 'c'; '0'; '1'; '2'; '3'; '4'; '5'; '6'; '7'; '8'; '9'; 'A'; 'B'; 'D'; 'E'; 'F'; 'G'; 'H'; 'I'; 'J'; 'K'; 'L'; 'M'; 'N'; 'O'; 'P'; 'Q'; 'R'; 'S'; 'T'; 'U'; 'W'; 'X'; 'Y'; 'Z']  dspbaimage=dspba_prim_channel_tall.svg  text=fprintf('Out%s', AdvDSPBChannelOutDisplay(latency));  style=Optimised  dataSignals=3  foldingEnabled=off  channels=1  sampleRate=200  packetBeginPresent=off  packetBeginEnabled=off  visibilities=dspba_ChannelOutVis(gcb)  latency=2  latencyCorrection=0  version=20211214
  CmpEQ : DSPBAPrim/CmpEQ  primtype=cmpeq  nInputs=2  nOutputs=1  omode=boolean  otype=sfix(16)  scale=2^-15  rndmethod=Unbiased  factor=1  satmethod=Symmetric  shift_vec=[0 1 2 -1]  value=0  inPortNames=[' '; ' ';]  outPortNames=[' ']  dspbaimage=dspba_prim.svg  text=fprintf('==');  style=Optimised  visibilities=0  advOptions=[]  version=20211007
  CmpGE : DSPBAPrim/CmpGE  primtype=cmpgte  nInputs=2  nOutputs=1  omode=boolean  otype=sfix(16)  scale=2^-15  rndmethod=Unbiased  factor=1  satmethod=Symmetric  shift_vec=[0 1 2 -1]  value=0  inPortNames=['a'; 'b';]  outPortNames=[' ']  dspbaimage=dspba_prim.svg  text=fprintf('a>=b');  style=Optimised  visibilities=0  advOptions=[]  version=20211007
  CmpLT : DSPBAPrim/CmpLT  primtype=cmplt  nInputs=2  nOutputs=1  omode=boolean  otype=sfix(16)  scale=2^-15  rndmethod=Unbiased  factor=1  satmethod=Symmetric  shift_vec=[0 1 2 -1]  value=0  inPortNames=['a'; 'b';]  outPortNames=[' ']  dspbaimage=dspba_prim.svg  text=fprintf('a<b');  style=Optimised  visibilities=0  advOptions=[]  version=20211007
  Const2 : DSPBAPrim/Const  primtype=const  nInputs=0  nOutputs=1  omode=Specify via dialog  otype=ufix(1)  scale=2^-0  rndmethod=Unbiased  factor=1  satmethod=Symmetric  shift_vec=[0 1 2 -1]  value=0  inPortNames=['+'; '+';]  outPortNames=[' ']  dspbaimage=dspba_prim.svg  text=fprintf('%s', num2str(value));  style=Optimised  visibilities=8 + 1024  floatPrecision=float32_m23  warnSaturation=on  version=20211007  SampleTime=inf
  Counter : DSPBAPrim/Counter  primtype=counter  nInputs=1  nOutputs=1  omode=Inherit via internal rule  otype=ufix(16)  scale=2^-0  rndmethod=Unbiased  factor=1  satmethod=Symmetric  shift_vec=[0 1 2 -1]  value=[prach.Nfft-1 prach.Nfft 1]  inPortNames=[' '; ' ';]  outPortNames=[' ']  dspbaimage=dspba_prim.svg  text=fprintf('counter\n[%d %d %d]', value(1), value(2), value(3));  style=Optimised  visibilities=8 + 1024  version=20211007
  Mux : DSPBAPrim/Mux  primtype=mux  nInputs=evalAionMaskParam(gcb,'value',1)+1  nOutputs=1  omode=Inherit via internal rule  otype=sfix(16)  scale=2^-15  rndmethod=Unbiased  factor=1  satmethod=Symmetric  shift_vec=[0 1 2 -1]  value=4  inPortNames=['s '; 'd0'; 'd1'; 'd2'; 'd3'; 'd4'; 'd5'; 'd6'; 'd7'; 'd8'; 'd9';]  outPortNames=[' ']  dspbaimage=dspba_prim_tall.svg  text=fprintf('%s', primtype);  style=Optimised  visibilities=1032  version=20211007
  SynthesisInfo : DSPBAPrim/SynthesisInfo  primtype=synthinfo  nInputs=0  nOutputs=0  omode=Inherit via internal rule  otype=sfix(16)  scale=2^-15  rndmethod=Truncate  factor=1  satmethod=Symmetric  shift_vec=[0 1 2 -1]  value=99  inPortNames=[' '; ' ';]  outPortNames=[' ']  dspbaimage=dspba_prim_ctrl.jpg  text=fprintf('Style=%s', style);  style=Scheduled  visibilities=2^17+2^18+2^19+2^20+2^21+2^22+2^23+2^24  constraintPair=None  constraintRelation=>  constraintLimit=2  modelRefSign=+  modelRef=''  showSchedule=off  simulationMode=Use Global Value  resetMinimization=Conditional - On for ChannelIn/Out only  version=20220106
  To Workspace12 : ToWorkspace  VariableName=prach_cout  SampleTime=-1
  To Workspace7 : ToWorkspace  VariableName=prach_vout  SampleTime=-1
  To Workspace8 : ToWorkspace  VariableName=prach_dout  SampleTime=-1
  Zero_insertion : Subsystem
  latch_0L : DSPBAControl/latch_0L
  dout : Outport  VectorParamsAs1DForOutWhenUnconnected=off
  vout : Outport  Port=2  VectorParamsAs1DForOutWhenUnconnected=off
  cout : Outport  Port=3  VectorParamsAs1DForOutWhenUnconnected=off
  TimeReference : Outport  Port=4  VectorParamsAs1DForOutWhenUnconnected=off
  ch_info : Outport  Port=5
  wires:
  ChannelIn/3 -> Zero_insertion/3(datain)
  Zero_insertion/2("chout ") -> Mux/1, ChannelOut/2
  Zero_insertion/1(valid_out) -> ChannelOut/1
  latch_0L/1 -> ChannelOut/4
  And1/1 -> latch_0L/1
  CmpEQ/1 -> And1/2
  Const2/1 -> CmpEQ/2
  ChannelIn/2 -> CmpEQ/1, Zero_insertion/2(chin)
  ChannelIn/4 -> latch_0L/2
  ChannelOut/4 -> TimeReference/1
  TimeRef/1 -> ChannelIn/4
  And/1 -> And1/1, Zero_insertion/1(valid_in)
  And2/1 -> And/2
  CmpLT/1 -> And2/2
  CmpGE/1 -> And2/1
  vin/1 -> ChannelIn/1
  chin/1 -> ChannelIn/2
  din/1 -> ChannelIn/3
  ChannelOut/3 -> dout/1, To Workspace8/1
  ChannelOut/2 -> cout/1, To Workspace12/1
  ChannelOut/1 -> vout/1, To Workspace7/1
  ChannelIn/1 -> Counter/1, And/1
  Counter/1 -> CmpGE/1, CmpLT/1
  ChannelIn/5 -> CmpGE/2
  ChannelIn/6 -> CmpLT/2
  prach_outstart/1 -> ChannelIn/5
  prach_outend/1 -> ChannelIn/6
  Zero_insertion/3(dataout) -> ChannelOut/3
  Mux/1 -> ChannelOut/5
  ChannelIn/7 -> Mux/2
  ChannelIn/8 -> Mux/3
  ChannelIn/9 -> Mux/4
  ChannelIn/10 -> Mux/5
  ChannelOut/5 -> ch_info/1
  ch0_info/1 -> ChannelIn/7
  ch1_info/1 -> ChannelIn/8
  ch2_info/1 -> ChannelIn/9
  ch3_info/1 -> ChannelIn/10

== system Lib_LongPRACH/Longprach_C_M_plane/LongPRACH_core/Timeref_capture_fifo ==
  valid_rd_in : Inport
  valid_wr_in : Inport  Port=2
  time_ref_in : Inport  Port=3
  channel_wr_in : Inport  Port=4
  ch_rd_in : Inport  Port=5
  And1 : DSPBAPrim/And  primtype=and  nInputs=2  nOutputs=1  omode=Inherit via internal rule  otype=sfix(16)  scale=2^-15  rndmethod=Unbiased  factor=1  satmethod=Symmetric  shift_vec=[0 1 2 -1]  value=0  inPortNames=[' '; ' '; ' '; ' '; ' '; ' '; ' '; ' '; ' '; ' '; ' '; ' '; ' '; ' '; ' '; ' '; ]  outPortNames=[' ']  dspbaimage=dspba_prim.svg  text=fprintf('&');  style=Optimised  visibilities=8+2  version=20211007
  CmpEQ1 : DSPBAPrim/CmpEQ  primtype=cmpeq  nInputs=2  nOutputs=1  omode=boolean  otype=sfix(16)  scale=2^-15  rndmethod=Unbiased  factor=1  satmethod=Symmetric  shift_vec=[0 1 2 -1]  value=0  inPortNames=[' '; ' ';]  outPortNames=[' ']  dspbaimage=dspba_prim.svg  text=fprintf('==');  style=Optimised  visibilities=0  advOptions=[]  version=20211007
  Const1 : DSPBAPrim/Const  primtype=const  nInputs=0  nOutputs=1  omode=Inherit via internal rule  otype=sfix(16)  scale=2^-15  rndmethod=Unbiased  factor=1  satmethod=Symmetric  shift_vec=[0 1 2 -1]  value=0  inPortNames=['+'; '+';]  outPortNames=[' ']  dspbaimage=dspba_prim.svg  text=fprintf('%s', num2str(value));  style=Optimised  visibilities=8 + 1024 + 2^18 + 2^20  floatPrecision=float32_m23  warnSaturation=on  version=20211007  SampleTime=inf
  FIFO : DSPBAPrim/FIFO  primtype=fifo  nInputs=3  nOutputs=4  omode=Inherit via internal rule  otype=sfix(16)  scale=2^-15  rndmethod=Unbiased  factor=1  satmethod=Symmetric  shift_vec=[0 1 2 -1]  value=[32 4 16]  inPortNames=['w'; 'd'; 'r'; 'f']  outPortNames=['v'; 'q'; 't'; 'f']  dspbaimage=dspba_prim_tall.svg  text=fprintf('fifo');  style=Optimised  visibilities=263168  version=20211007  user_sclr=off
  GPIn : DSPBAPrim/GPIn  primtype=gpin  nInputs=evalAionMaskParam(gcb,'value',1)  nOutputs=evalAionMaskParam(gcb,'value',1)  omode=Inherit via internal rule  otype=sfix(16)  scale=2^-15  rndmethod=Unbiased  factor=1  satmethod=Symmetric  shift_vec=[0 1 2 -1]  value=5  inPortNames=[' ' ' ' ' ' ' ' ' ' ' ' ' ' ' ' ' ' ' ' ' ' ' ' ' ' ' ' ' ' ' ' ' ' ' ' ' ' ' ' ' ' ' ' ' ' ' ' ' ' ' ' ' ' ' ' ' ' ' ' ' ' ' ' ' ' ' ' ' ']'  outPortNames=[' ' ' ' ' ' ' ' ' ' ' ' ' ' ' ' ' ' ' ' ' ' ' ' ' ' ' ' ' ' ' ' ' ' ' ' ' ' ' ' ' ' ' ' ' ' ' ' ' ' ' ' ' ' ' ' ' ' ' ' ' ' ' ' ' ' ' ' ' ']'  dspbaimage=dspba_prim_channel_tall.svg  text=fprintf('GPIn%s', AdvDSPBInDisplay(latencyCorrection));  style=Optimised  visibilities=1024  latencyCorrection=0  scheduleOrigin=on  version=20211214
  GPOut : DSPBAPrim/GPOut  primtype=gpout  nInputs=evalAionMaskParam(gcb,'value',1)  nOutputs=evalAionMaskParam(gcb,'value',1)  omode=Inherit via internal rule  otype=sfix(16)  scale=2^-15  rndmethod=Unbiased  factor=1  satmethod=Symmetric  shift_vec=[0 1 2 -1]  value=1  inPortNames=[' ' ' ' ' ' ' ' ' ' ' ' ' ' ' ' ' ' ' ' ' ' ' ' ' ' ' ' ' ' ' ' ' ' ' ' ' ' ' ' ' ' ' ' ' ' ' ' ' ' ' ' ' ' ' ' ' ' ' ' ' ' ' ' ' ' ' ' ' ']'  outPortNames=[' ' ' ' ' ' ' ' ' ' ' ' ' ' ' ' ' ' ' ' ' ' ' ' ' ' ' ' ' ' ' ' ' ' ' ' ' ' ' ' ' ' ' ' ' ' ' ' ' ' ' ' ' ' ' ' ' ' ' ' ' ' ' ' ' ' ' ' ' ']'  dspbaimage=dspba_prim_channel_tall.svg  text=fprintf('GPOut%s', AdvDSPBOutDisplay(latency, latencyCorrection));  style=Optimised  visibilities=1024  latency=1  latencyCorrection=0  version=20211214
  SynthesisInfo : DSPBAPrim/SynthesisInfo  primtype=synthinfo  nInputs=0  nOutputs=0  omode=Inherit via internal rule  otype=sfix(16)  scale=2^-15  rndmethod=Truncate  factor=1  satmethod=Symmetric  shift_vec=[0 1 2 -1]  value=99  inPortNames=[' '; ' ';]  outPortNames=[' ']  dspbaimage=dspba_prim_ctrl.jpg  text=fprintf('Style=%s', style);  style=Scheduled  visibilities=2^17+2^18+2^19+2^20+2^21+2^22+2^23+2^24  constraintPair=None  constraintRelation=>  constraintLimit=2  modelRefSign=+  modelRef=''  showSchedule=off  simulationMode=Use Global Value  resetMinimization=Conditional - On for ChannelIn/Out only  version=20220106
  Terminator : Terminator
  Terminator1 : Terminator
  Terminator2 : Terminator
  latch_0L : DSPBAControl/latch_0L
  rising_edge : Subsystem
  rising_edge1 : Subsystem
  time_ref_out : Outport
  wires:
  latch_0L/1 -> GPOut/1
  FIFO/2 -> latch_0L/2
  valid_rd_in/1 -> GPIn/1
  GPIn/3 -> FIFO/2
  GPIn/2 -> rising_edge/1(In1)
  rising_edge1/1(Out1) -> And1/2
  GPIn/1 -> rising_edge1/1(In1)
  channel_wr_in/1 -> GPIn/4
  CmpEQ1/1 -> And1/1
  GPIn/5 -> CmpEQ1/1
  And1/1 -> FIFO/3, latch_0L/1
  time_ref_in/1 -> GPIn/3
  Const1/1 -> CmpEQ1/2
  valid_wr_in/1 -> GPIn/2
  ch_rd_in/1 -> GPIn/5
  FIFO/3 -> Terminator1/1
  GPOut/1 -> time_ref_out/1
  rising_edge/1(Out1) -> FIFO/1
  FIFO/4 -> Terminator2/1
  FIFO/1 -> Terminator/1
